simulink model "Openloop_DC_motor_offline2"  (R2022a)
settings: Solver=FixedStepAuto  StartTime=0.0  StopTime=2  FixedStep=1e-6  RelTol=1e-3
InitFcn:
  | Ts = 1e-4;
libraries: spsIGBTDiodeLib x4, spsSeriesRLCBranchLib x2, spsDCVoltageSourceLib x2, spsDCMachineLib x1, simulink x1, spspowerguiLib x1
settings Model: Creator=XCY  LastModifiedBy=Administrator
settings SolverCC: AlgebraicLoopSolver=TrustRegion
settings DataIOCC: ReturnWorkspaceOutputs=off
settings DebuggingCC: UnconnectedInputMsg=warning  UnconnectedOutputMsg=warning  UnconnectedLineMsg=warning  SFMachineParentedDataDiag=warning  ArithmeticOperatorsInVariantConditions=warning
settings SFSimCC: SimUseLocalCustomCode=off  CustomCodeUndefinedFunction=UseInterfaceOnly
settings RTWCC: RTWUseLocalCustomCode=off
settings CodeAppCC: StateflowObjectComments=on
settings SimscapeCC: SimscapeNormalizeSystem=off

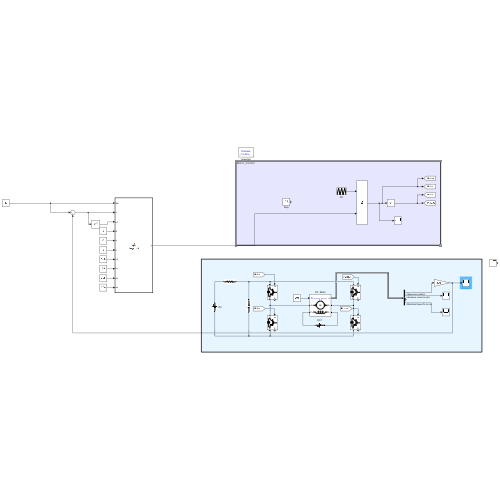
[thumbnail: Simulink's stored preview of the top-level diagram]
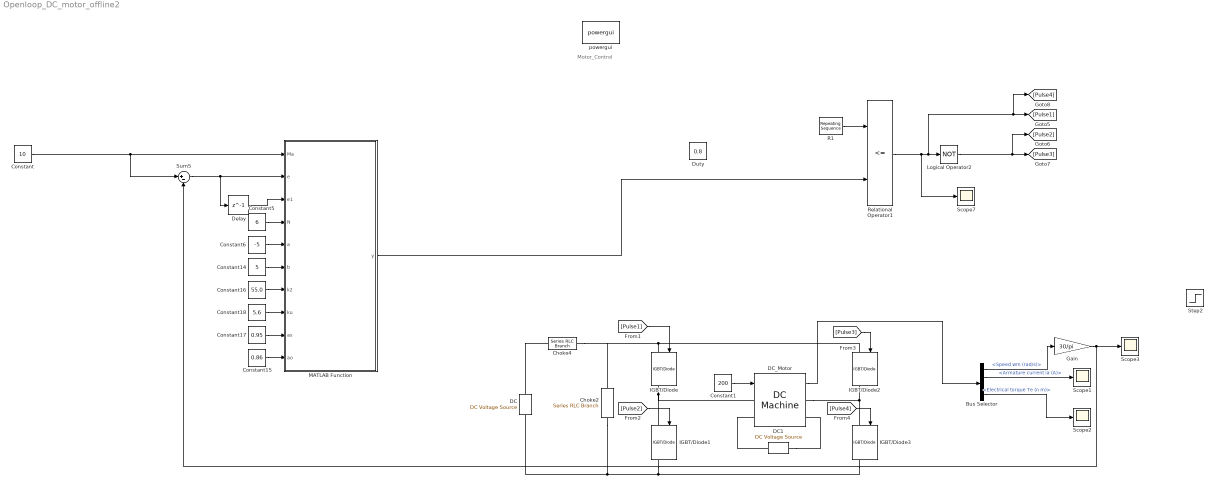
== system Openloop_DC_motor_offline2 ==
  note: Motor_Control
  Bus Selector : BusSelector  OutputSignals=Speed wm (rad/s),Armature current ia (A),Field current if (A),Electrical torque Te (n m)
  Choke2 : spsSeriesRLCBranchLib/Series RLC Branch  LConnTagsString=__new0  RConnTagsString=__new0  BranchType=C  Resistance=5e-3  Inductance=2e-3  SetiL0=off  InitialCurrent=0  Capacitance=1e-6  Setx0=off  InitialVoltage=0  Measurements=None
  Choke4 : spsSeriesRLCBranchLib/Series RLC Branch  LConnTagsString=__new0  RConnTagsString=__new0  BranchType=R  Resistance=5e-3  Inductance=2e-3  SetiL0=off  InitialCurrent=0  Capacitance=1e-6  Setx0=off  InitialVoltage=0  Measurements=None
  Constant : Constant  Value=10
  Constant1 : Constant  Value=200
  Constant14 : Constant  Value=5  OutDataTypeStr=Inherit: Inherit via back propagation
  Constant15 : Constant  Value=0.86  OutDataTypeStr=Inherit: Inherit via back propagation
  Constant16 : Constant  Value=55.0  OutDataTypeStr=Inherit: Inherit via back propagation
  Constant17 : Constant  Value=0.95  OutDataTypeStr=Inherit: Inherit via back propagation
  Constant18 : Constant  Value=5.6  OutDataTypeStr=Inherit: Inherit via back propagation
  Constant5 : Constant  Value=6  OutDataTypeStr=Inherit: Inherit via back propagation
  Constant6 : Constant  Value=-5
  DC : spsDCVoltageSourceLib/DC Voltage Source  Amplitude=600  Measurements=None
  DC1 : spsDCVoltageSourceLib/DC Voltage Source  Amplitude=240  Measurements=None
  DC_Motor : spsDCMachineLib/DC Machine  PresetModel=No  MechanicalLoad=Torque TL  FieldType=Wound  ShowDetailedParameters=on  MeasurementBus=off  RLa="[ 0.6  0.012]"  RLf="[ 240  120]"  Laf=1.8  MachineConstant=Torque constant (N.m/A)  Ke=1.8  Kt=1.8  J=1  Bm=0.1  Tf=0  w0=0  Ifinit=1  TsPowergui=0  TsBlock=-1
      settings: AttributesFormatString=\n
  Delay : Delay  DelayLength=1
  Duty : Constant  Value=0.8
  Gain : Gain  Gain=30/pi
  IGBT/Diode{,1..3} (4 alike) : spsIGBTDiodeLib/IGBT//Diode  Ron=1e-3  Rs=1e5  Cs=inf  Measurements=on
  Logical Operator2 : Logic  Operator=NOT  AllPortsSameDT=off  OutDataTypeStr=boolean
  MATLAB Function : MATLAB Function  TreatAsAtomicUnit=on
      settings: MinAlgLoopOccurrences=on
  R1 : simulink/Sources/Repeating Sequence  rep_seq_t=[0 0.00005 0.0001]  rep_seq_y=[0 1 0]
  Relational Operator1 : RelationalOperator  Operator=<=  OutDataTypeStr=boolean  RndMeth=Simplest  InputSameDT=off
  Scope{1..3,7} (4 alike) : Scope
  Step2 : Step  Time=1.5  After=200  SampleTime=0
  Sum5 : Sum  Inputs=|+-
  powergui : spspowerguiLib/powergui  Priority=1  SimulationMode=Discrete  SampleTime=1e-6  frequency=60  Iterations=50  frequencyindice=0  Pbase=100e6  ErrMax=1e-4  UnitsV=kV  UnitsW=MW  buscounter=0  FunctionMessages=off  echomessages=off  EnableUseOfTLC=off  CurrentSourceSwitches=off  DisableSnubberDevices=off  DisableRonSwitches=off  DisableVfSwitches=off  DisplayEquations=off  AutomaticDiscreteSolvers=off  SolverType=Tustin/Backward Euler (TBE)  Interpol=off  ExternalGateDelay=off  methode=off  Ts=100  x0status=blocks  SPID=off  SwTol=0  HookPort=off  NonlinearTolerance=1e-4  nMaxIteration=100  ContinueOnMaxIteration=off  RestoreLinks=warning  ResistiveCurrentMeasurement=off  Frange=[0:2:500]  Ylog=off  Xlog=on  ShowGrid=off  save=off  variable=ZData  structure=0  ZoomFFT=off  StartTime=0.0  cycles=1  DisplayStyle=1  fundamental=60  FreqAxis=off  MaxFrequency=1000  frequencyindicesteady=1  RmsSteady=1  display=off
  wires:
  Bus Selector/2 -> Scope1/1  "<Armature current ia (A)>"
  Bus Selector/4 -> Scope2/1  "<Electrical torque Te (n m)>"
  Bus Selector/1 -> Gain/1  "<Speed wm (rad/s)>"
  [Pulse1] -> IGBT/Diode/1
  [Pulse2] -> IGBT/Diode1/1
  Gain/1 -> Sum5/2, Scope3/1
  DC_Motor/1 -> Bus Selector/1
  [Pulse3] -> IGBT/Diode2/1
  [Pulse4] -> IGBT/Diode3/1
  Constant1/1 -> DC_Motor/1
  Relational Operator1/1 -> Logical Operator2/1, [Pulse1], [Pulse4], Scope7/1
  Logical Operator2/1 -> [Pulse3], [Pulse2]
  R1/1 -> Relational Operator1/1
  MATLAB Function/1(y) -> Relational Operator1/2
  Delay/1 -> MATLAB Function/3(e1)
  Constant/1 -> MATLAB Function/1(Ma), Sum5/1
  Constant18/1 -> MATLAB Function/8(ku)
  Constant17/1 -> MATLAB Function/9(as)
  Constant5/1 -> MATLAB Function/4(N)
  Constant16/1 -> MATLAB Function/7(k2)
  Constant14/1 -> MATLAB Function/6(b)
  Constant6/1 -> MATLAB Function/5(a)
  Constant15/1 -> MATLAB Function/10(ao)
  Sum5/1 -> Delay/1, MATLAB Function/2(e)
  connections:
  IGBT/Diode1/RConn1 -- IGBT/Diode3/RConn1 -- Choke2/RConn1 -- DC/LConn1
  DC1/LConn1 -- DC_Motor/RConn2
  IGBT/Diode/LConn1 -- Choke4/RConn1 -- Choke2/LConn1 -- IGBT/Diode2/LConn1
  DC1/RConn1 -- DC_Motor/LConn2
  IGBT/Diode3/LConn1 -- DC_Motor/RConn1 -- IGBT/Diode2/RConn1
  IGBT/Diode/RConn1 -- DC_Motor/LConn1 -- IGBT/Diode1/LConn1
  DC/RConn1 -- Choke4/LConn1

== matlab function Openloop_DC_motor_offline2/MATLAB Function ==
  data: Ma input; e input; e1 input; N input; y output; a input; b input; k2 input; ku input; as input; ao input
function y = fuzyy_pid(Ma,e,e1,N,a,b,k2,ku,as,ao)


	ed = e - e1;
	E = -(2 * N) * (e * k2 - (a + b)) / (b - a);    
	E1 = E;
	EC = -(2 * N) * (ed - (a + b)) / (b - a);
	EC1 = 270 * EC;
	a1 = (1 / N) * (as - ao) * abs(E1) + ao;
	y1 = (-(a1 * E1 + (1 - a1) * EC1) / 2);
    y2=y1*ku;
    y=y2*Ma;
    
end
